simulink model "PSS2B_fmu_RaPId"  (R2020a)
settings: Solver=FixedStepAuto  StartTime=0.0  StopTime=5  FixedStep=0.005  RelTol=1e-2
libraries: fmu_me_lib x1
settings Model: Creator=meagh  LastModifiedBy=meagh

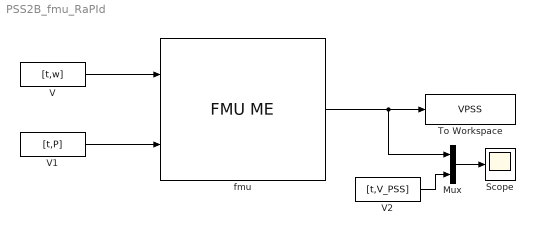
== system PSS2B_fmu_RaPId ==
  Mux : Mux  Inputs=2
  Scope : Scope
  To Workspace : ToWorkspace  VariableName=VPSS  SaveFormat=Timeseries  SampleTime=-1
  V : FromWorkspace  VariableName=[t,w]
  V1 : FromWorkspace  VariableName=[t,P]
  V2 : FromWorkspace  VariableName=[t,V_PSS]
  fmu : fmu_me_lib/FMU ME  Description=Simulates an FMU for Model Exchange 1.0 or Model Exchange 2.0.  dummy=0
  wires:
  V/1 -> fmu/1
  V1/1 -> fmu/2
  fmu/1 -> Mux/1, To Workspace/1
  Mux/1 -> Scope/1
  V2/1 -> Mux/2
